simulink model "cMu"  (R2015a)
settings: Solver=ode45  StartTime=0.0  StopTime=(N-1)/Fs  MaxStep=1/Fs  MinStep=1/Fs  RelTol=1e-3  AbsTol=1/Fs
undefined symbols (not defined in the file): Fs
libraries: commsrccod2 x2
settings Model: Creator=Javi  LastModifiedBy=Javi
settings SolverCC: InitialStep=1/Fs

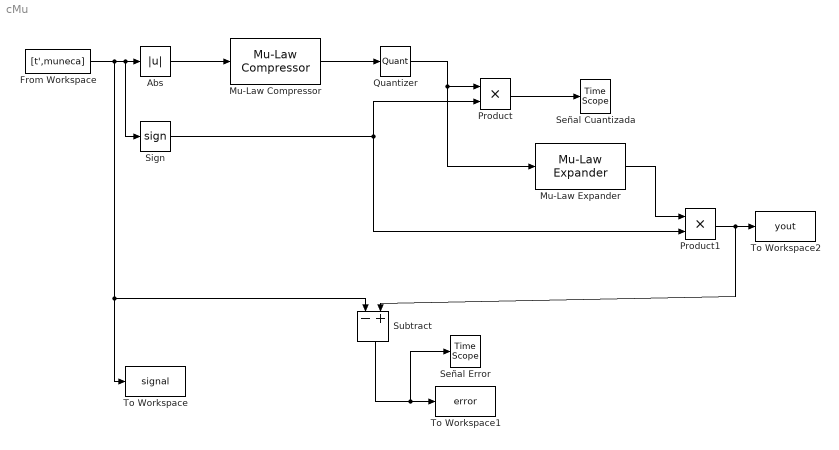
== system cMu ==
  Abs : Abs
  From Workspace : FromWorkspace  VariableName=[t',muneca]  SampleTime=1/Fs
  Mu-Law Compressor : commsrccod2/Mu-Law Compressor  mu=255  V=2048
  Mu-Law Expander : commsrccod2/Mu-Law Expander  mu=255  V=2048
  Product : Product
  Product1 : Product
  Quantizer : Quantizer  QuantizationInterval=256  LinearizeAsGain=off
  Señal Cuantizada : TimeScope
  Señal Error : TimeScope
  Sign : Signum
  Subtract : Sum  Inputs=-+
  To Workspace : ToWorkspace  VariableName=signal  SampleTime=-1
      settings: Save2DSignal=2-D array (concatenate along first dimension)
  To Workspace1 : ToWorkspace  VariableName=error  SampleTime=-1
      settings: Save2DSignal=2-D array (concatenate along first dimension)
  "To Workspace2 " : ToWorkspace  VariableName=yout  SampleTime=-1
      settings: Save2DSignal=2-D array (concatenate along first dimension)
  wires:
  From Workspace/1 -> Sign/1, Abs/1, Subtract/1, To Workspace/1
  Subtract/1 -> Señal Error/1, To Workspace1/1
  Abs/1 -> Mu-Law Compressor/1
  Mu-Law Compressor/1 -> Quantizer/1
  Product/1 -> Señal Cuantizada/1
  Quantizer/1 -> Mu-Law Expander/1, Product/1
  Mu-Law Expander/1 -> Product1/1
  Sign/1 -> Product1/2, Product/2
  Product1/1 -> Subtract/2, "To Workspace2 "/1
